simulink model "receiveBuffer"  (R2015a)
settings: Solver=FixedStepDiscrete  StartTime=0.0  StopTime=25  FixedStep=1  RelTol=1e-3
undefined symbols (not defined in the file or in its folder): sigbuilder_block
settings Model: Creator=qiji  LastModifiedBy=qiji
settings OptimizationCC: BlockReduction=off  ConditionallyExecuteInputs=off
settings DebuggingCC: UnderspecifiedInitializationDetection=Classic  MergeDetectMultiDrivingBlocksExec=none  SolverPrmCheckMsg=warning  SingleTaskRateTransMsg=error

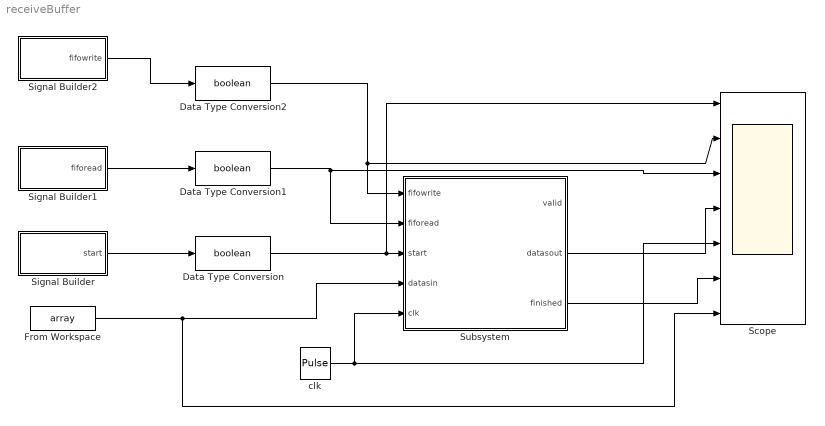
== system receiveBuffer ==
  Data Type Conversion : DataTypeConversion  OutDataTypeStr=boolean
  Data Type Conversion1 : DataTypeConversion  OutDataTypeStr=boolean
  Data Type Conversion2 : DataTypeConversion  OutDataTypeStr=boolean
  From Workspace : FromWorkspace  VariableName=array  SampleTime=0
  Scope : Scope  NumInputPorts=7
      settings: YMin=-5~-5~-5~-5~-5~-5~-5  YMax=5~5~5~5~5~5~5  MaxDataPoints=5000000
  Signal Builder : Subsystem  Tag=STV Subsys  LoadFcn=sigbuilder_block('load');  StartFcn=sigbuilder_block('start');  StopFcn=sigbuilder_block('stop');  ClipboardFcn=sigbuilder_block('clipboard');  mask(Sigbuilder block){}
      mask help: Simulink:masks:SigbuilderBlock_MD
      mask init:
      | if ~strcmp(get_param(bdroot(gcbh),'SimulationStatus'),'stopped') tuvar = sigbuilder_block('maskInit'); end
      settings: CopyFcn=sigbuilder_block('copy');  DeleteFcn=sigbuilder_block('delete');  ModelCloseFcn=sigbuilder_block('modelClose');  PreSaveFcn=sigbuilder_block('preSave');  PauseFcn=sigbuilder_block('pause');  ContinueFcn=sigbuilder_block('continue');  NameChangeFcn=sigbuilder_block('namechange');  OpenFcn=sigbuilder_block('open',[408 61.5 550.5 399.75 ]);  CloseFcn=sigbuilder_block('close');
      mask Display: plot(0, 0, 100, 100,[2, 2, 32, 32, 2], [68, 8, 8, 68, 68],[32, 2], [38, 38], [32, 19, 2],[53, 60, 44], [32, 17, 17, 2],[16, 16, 31, 31]);txt = getActiveGroup(gcbh);text(2, 100, txt,'verticalAlignment', 'top');
  Signal Builder1 : Subsystem  Tag=STV Subsys  LoadFcn=sigbuilder_block('load');  StartFcn=sigbuilder_block('start');  StopFcn=sigbuilder_block('stop');  ClipboardFcn=sigbuilder_block('clipboard');  mask(Sigbuilder block){}
      mask help: Simulink:masks:SigbuilderBlock_MD
      mask init:
      | if ~strcmp(get_param(bdroot(gcbh),'SimulationStatus'),'stopped') tuvar = sigbuilder_block('maskInit'); end
      settings: CopyFcn=sigbuilder_block('copy');  DeleteFcn=sigbuilder_block('delete');  ModelCloseFcn=sigbuilder_block('modelClose');  PreSaveFcn=sigbuilder_block('preSave');  PauseFcn=sigbuilder_block('pause');  ContinueFcn=sigbuilder_block('continue');  NameChangeFcn=sigbuilder_block('namechange');  OpenFcn=sigbuilder_block('open',[408 61.5 550.5 399.75 ]);  CloseFcn=sigbuilder_block('close');
      mask Display: plot(0, 0, 100, 100,[2, 2, 32, 32, 2], [68, 8, 8, 68, 68],[32, 2], [38, 38], [32, 19, 2],[53, 60, 44], [32, 17, 17, 2],[16, 16, 31, 31]);txt = getActiveGroup(gcbh);text(2, 100, txt,'verticalAlignment', 'top');
  Signal Builder2 : Subsystem  Tag=STV Subsys  LoadFcn=sigbuilder_block('load');  StartFcn=sigbuilder_block('start');  StopFcn=sigbuilder_block('stop');  ClipboardFcn=sigbuilder_block('clipboard');  mask(Sigbuilder block){}
      mask help: Simulink:masks:SigbuilderBlock_MD
      mask init:
      | if ~strcmp(get_param(bdroot(gcbh),'SimulationStatus'),'stopped') tuvar = sigbuilder_block('maskInit'); end
      settings: CopyFcn=sigbuilder_block('copy');  DeleteFcn=sigbuilder_block('delete');  ModelCloseFcn=sigbuilder_block('modelClose');  PreSaveFcn=sigbuilder_block('preSave');  PauseFcn=sigbuilder_block('pause');  ContinueFcn=sigbuilder_block('continue');  NameChangeFcn=sigbuilder_block('namechange');  OpenFcn=sigbuilder_block('open',[408 61.5 550.5 399.75 ]);  CloseFcn=sigbuilder_block('close');
      mask Display: plot(0, 0, 100, 100,[2, 2, 32, 32, 2], [68, 8, 8, 68, 68],[32, 2], [38, 38], [32, 19, 2],[53, 60, 44], [32, 17, 17, 2],[16, 16, 31, 31]);txt = getActiveGroup(gcbh);text(2, 100, txt,'verticalAlignment', 'top');
  Subsystem : Subsystem
  clk : DiscretePulseGenerator  PulseType=Time based  Amplitude=true  PulseWidth=50
  wires:
  clk/1 -> Scope/5, Subsystem/5(clk)
  Subsystem/2(datasout) -> Scope/4
  Signal Builder/1(start) -> Data Type Conversion/1
  Data Type Conversion/1 -> Scope/1, Subsystem/3(start)
  Signal Builder1/1(fiforead) -> Data Type Conversion1/1
  Data Type Conversion1/1 -> Scope/3, Subsystem/2(fiforead)
  Signal Builder2/1(fifowrite) -> Data Type Conversion2/1
  Data Type Conversion2/1 -> Subsystem/1(fifowrite), Scope/2
  From Workspace/1 -> Scope/7, Subsystem/4(datasin)
  Subsystem/3(finished) -> Scope/6

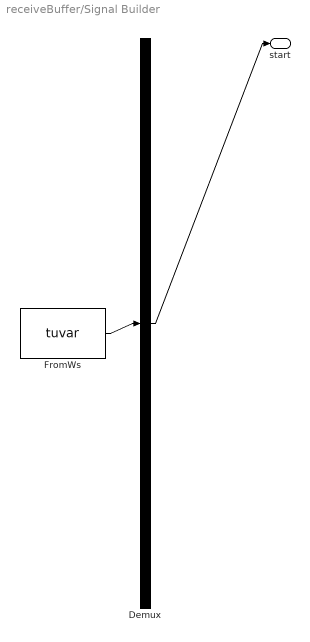
== system receiveBuffer/Signal Builder ==
  Demux : Demux  Tag=STV Demux  Outputs=1
  FromWs : FromWorkspace  Tag=STV FromWs  VariableName=tuvar  SampleTime=0  OutputAfterFinalValue=Setting to zero
      SigBuilderData=|
      | common.afterFinalStr = 'Set to zero'
      | common.sampleTime = '0'
      | dataSet.timeRange = [0 20]
      | dataSet.name = 'Group 1'
      | sbobj.Groups.Name = 'Group 1'
      | sbobj.Groups.Signals.Name = 'start'
      | sbobj.Groups.Signals.XData = [0 2 2 3.95 3.95 20]
      | sbobj.Groups.Signals.YData = [0 0 1 1 0 0]
      | sbobj.Groups.TimeRange = [0 20]
  start : Outport  Tag=STV Outport
  wires:
  Demux/1 -> start/1
  FromWs/1 -> Demux/1

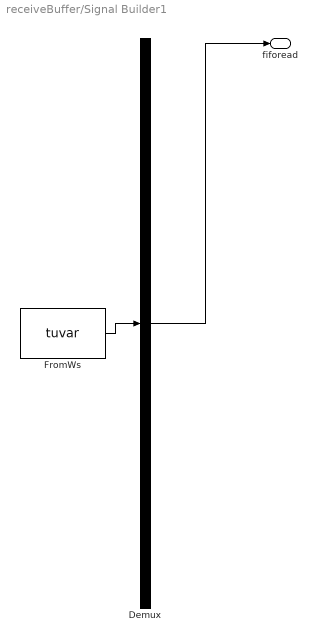
== system receiveBuffer/Signal Builder1 ==
  Demux : Demux  Tag=STV Demux  Outputs=1
  FromWs : FromWorkspace  Tag=STV FromWs  VariableName=tuvar  SampleTime=0
      SigBuilderData=|
      | common.afterFinalStr = 'Extrapolate'
      | common.sampleTime = 0
      | dataSet.timeRange = [0 20]
      | dataSet.name = 'Group 1'
      | sbobj.Groups.Name = 'Group 1'
      | sbobj.Groups.Signals.Name = 'fiforead'
      | sbobj.Groups.Signals.XData = [0 14 14 20]
      | sbobj.Groups.Signals.YData = [0 0 1 1]
      | sbobj.Groups.TimeRange = [0 20]
  fiforead : Outport  Tag=STV Outport
  wires:
  FromWs/1 -> Demux/1
  Demux/1 -> fiforead/1

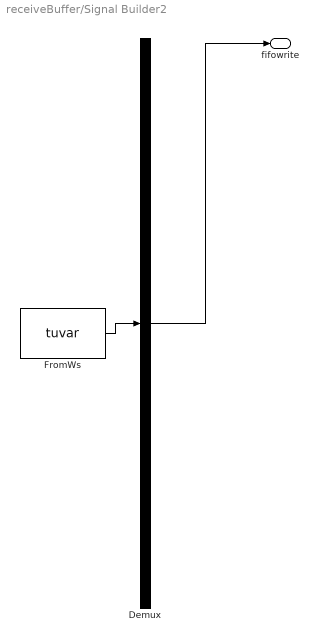
== system receiveBuffer/Signal Builder2 ==
  Demux : Demux  Tag=STV Demux  Outputs=1
  FromWs : FromWorkspace  Tag=STV FromWs  VariableName=tuvar  SampleTime=0
      SigBuilderData=|
      | common.afterFinalStr = 'Extrapolate'
      | common.sampleTime = 0
      | dataSet.timeRange = [0 20]
      | dataSet.name = 'Group 1'
      | sbobj.Groups.Name = 'Group 1'
      | sbobj.Groups.Signals.Name = 'fifowrite'
      | sbobj.Groups.Signals.XData = [0 5 5 13 13 20]
      | sbobj.Groups.Signals.YData = [0 0 1 1 0 0]
      | sbobj.Groups.TimeRange = [0 20]
  fifowrite : Outport  Tag=STV Outport
  wires:
  Demux/1 -> fifowrite/1
  FromWs/1 -> Demux/1

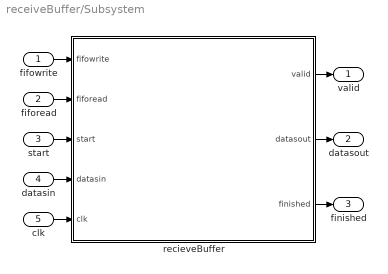
== system receiveBuffer/Subsystem ==
  fifowrite : Inport
  fiforead : Inport  Port=2
  start : Inport  Port=3
  datasin : Inport  Port=4
  clk : Inport  Port=5
  recieveBuffer : Stateflow chart  TreatAsAtomicUnit=on
  valid : Outport
  datasout : Outport  Port=2
  finished : Outport  Port=3
  wires:
  recieveBuffer/2(datasout) -> datasout/1
  recieveBuffer/3(finished) -> finished/1
  fifowrite/1 -> recieveBuffer/1(fifowrite)
  fiforead/1 -> recieveBuffer/2(fiforead)
  start/1 -> recieveBuffer/3(start)
  clk/1 -> recieveBuffer/5(clk)
  datasin/1 -> recieveBuffer/4(datasin)
  recieveBuffer/1(valid) -> valid/1

== stateflow chart receiveBuffer/Subsystem/recieveBuffer ==
  settings: executeAtInitialization=1  initializeOutput=1
  state judge [function]
    (default) -> (junction 54)
    (junction 40) -> (junction 39) [order 1] : [fifowrite==true]
    (junction 54) -> (junction 40) [order 2] : [start==false]
    (junction 39) -> (junction 17)
    (junction 40) -> (junction 23) [order 2]
    (junction 54) -> (junction 57) [order 1] : [start==true]
        | {
        | tail=uint8(1);
        | head=uint8(1);
        | readtag=false;
        | valid=false;
        | finished=false;
        | datasout=zero;
        | }
    (junction 23) -> (junction 21) [order 1] : [fiforead==true]
    (junction 17) -> (junction 19) [order 1] : [tail==17]
    (junction 23) -> (junction 20) [order 2] : {
        | valid=false;
        | finished=false;
        | datasout=zero;
        | }
    (junction 21) -> (junction 14)
    (junction 17) -> (junction 18) [order 2] : {
        | fifo(:, tail)=datasin;
        | tail=tail+1;
        | }
    (junction 19) -> (junction 5) : {tail=uint8(1)}
    (junction 14) -> (junction 11) [order 1] : [head==tail]
    (junction 14) -> (junction 9) [order 2] : {
        | finished=false;
        | valid=true;
        | datasout=fifo(:, head);
        | head=head+1;
        | }
    (junction 11) -> (junction 8) : {
        | head=uint8(1);
        | tail=uint8(1);
        | readtag=false;
        | finished=true;
        | valid=false;
        | datasout=zero;
        | }
    (junction 5) -> (junction 18)
    (junction 18) -> (junction 38) : {
        | valid=false;
        | finished=false;
        | datasout=zero;
        | }
    (junction 8) -> (junction 9)
    (junction 9) -> (junction 12)
    (junction 38) -> (junction 20)
    (junction 12) -> (junction 20)
    (junction 20) -> (junction 55)
    (junction 55) -> (junction 57)
  state start
    start -> start : [clk==1]
        | {
        | judge();
        | }
  (default) -> start : {
      | zero=[false; false;false;false;false; false; false; false;...
      |  false; false; false; false; false; false; false; false]
      | }
  data: fifowrite input boolean; fiforead input boolean; start input boolean; datasin input boolean size=16; valid output boolean; datasout output boolean size=16; finished output boolean; head local uint8; tail local uint8; readtag local boolean; zero local boolean size=16 =[0,0,0,0,0,0,0,0,0,0,0,0,0,0,0,0]; clk input boolean; fifo local boolean size=16,16
  data valid settings: description=数据有效信号，配合datasout使用
  data datasout settings: description=向上层提交数据时的数据线，当vailid=1时数据线上的数据有效
  data finished settings: description=当数据传递结束时，给出finished=1的信号
  data head settings: description=address of the quence head
  data tail settings: description=address of quence tail
  data readtag settings: description=the sample of reading data
